simulink model "SF018A_EotProtn"  (R2013b)
settings: Solver=FixedStepDiscrete  SolverMode=SingleTasking  StartTime=0.0  StopTime=0.002  FixedStep=.002  RelTol=1e-3
undefined symbols (not defined in the file): ALLSPDDAMPG_CNT_U08, ALLSPDGAIN_CNT_U08, ARCHGLBPRM_2MILLISEC_SEC_F32, DISTLPFILFRQ_HZ_F32, EOTDAMPGLOLIM_MOTNWTMTR_F32, EOTGAINHILIM_ULS_F32, EotProtnActvRegnBypMaxThd, EotProtnDampgSlew, EotProtnDampgVehSpdTbl, EotProtnDeltaTqThd, EotProtnDftPosn, EotProtnEntrGainVehSpdTbl, EotProtnEntrGainX, EotProtnEntrStLpFilFrq, EotProtnExitDampgY, EotProtnExitStLpFilFrq, EotProtnHwAgGain, EotProtnHwAgMax, EotProtnHwAgMin, EotProtnHwDegDampgX, EotProtnMotSpdIncptSca, EotProtnMotSpdIncptX, EotProtnMotSpdIncptY, EotProtnMotVelGain, EotProtnNormDampgY, EotProtnPosnRampStep, EotProtnRackTrvlLimrAuthyThd, EotProtnRackTrvlLimrAuthyThdLimd, EotProtnRackTrvlLimrEna, EotProtnRackTrvlLimrRng, EotProtnRackTrvlLimrRngLimd, EotProtnRackTrvlLimrVehSpdThd, EotProtnRunEotVelImpctAndSoftEndStop, EotProtnSoftEndStopAuthyThd, EotProtnSoftEndStopEna, EotProtnSoftEndStopVehSpdThd, FIRSTPTDAMPG_CNT_U08, LASTPTGAIN_CNT_U08, SOFTENDSTOPSTDI_CNT_U08, SOFTENDSTOPSTENTR_CNT_U08, SOFTENDSTOPSTEXIT_CNT_U08, SOFTENDSTOPSTNORM_CNT_U08, SYSGLBPRM_MOTTQCMDHILIM_MOTNWTMTR_F32, ZEROMOTTQCMD_MOTNWTMTR_F32
libraries: NxtrAbslt x16, FloatToFixd x14, FixdToFloat x6, Fil x5, NxtrLim x5, simulink x4, NxtrMax x4, LnrIntrpnDyn x3, NxtrSign x2, BilnrIntrpnMplXDyn x2, BilnrIntrpnMplX x1, LnrIntrpn x1
(part 5 of 5)

== system SF018A_EotProtn/EotProtn/EotProtnPer1/SoftEndStop/FildEotGain/If Action Subsystem4 ==
  In1 : Inport
  Action Port : ActionPort  ActionType=default
  CopyRight2 : Subsystem  Description=|  mask(Copyright Information){none=on}
      | Copyright info block.                                               
      |                                                                     
      | Place copyright information at the top of every subsystem in design.
      mask prompts: none "No parameters"
      mask help: Place copyright information at the top of every subsystem in design.
      mask Display:
      | NxtrConf = 'Nexteer Confidential';
      | 
      | sys = bdroot; %handle for the current model ("system")
      | first = get_param(sys,'Created');
      | if(isempty(first))
      |     first = datestr(now,'yyyy');
      | else
      |     first = first(end-3:end);  %year is last four digits
      | end
      | 
      | last = get_param(sys,'LastModifiedDate');
      | if isempty(last)
      |     last = datestr(now,'yyyy');
      | else
      |     last = last(end-3:end);
      | end
      | 
      | if strcmp(first,last)
      |     fprintf('%s -- Copyright %s Nexteer',NxtrConf,first)
      | else
      |     fprintf('%s -- %s%s- %s Nexteer',NxtrConf,char(169),first,last)
      | end
  Out1 : Outport
  wires:
  In1/1 -> Out1/1

== system SF018A_EotProtn/EotProtn/EotProtnPer1/SoftEndStop/FildEotGain/If Action Subsystem5 ==
  In1 : Inport
  Action Port : ActionPort  ActionType=case
  CopyRight2 : Subsystem  Description=|  mask(Copyright Information){none=on}
      | Copyright info block.                                               
      |                                                                     
      | Place copyright information at the top of every subsystem in design.
      mask prompts: none "No parameters"
      mask help: Place copyright information at the top of every subsystem in design.
      mask Display:
      | NxtrConf = 'Nexteer Confidential';
      | 
      | sys = bdroot; %handle for the current model ("system")
      | first = get_param(sys,'Created');
      | if(isempty(first))
      |     first = datestr(now,'yyyy');
      | else
      |     first = first(end-3:end);  %year is last four digits
      | end
      | 
      | last = get_param(sys,'LastModifiedDate');
      | if isempty(last)
      |     last = datestr(now,'yyyy');
      | else
      |     last = last(end-3:end);
      | end
      | 
      | if strcmp(first,last)
      |     fprintf('%s -- Copyright %s Nexteer',NxtrConf,first)
      | else
      |     fprintf('%s -- %s%s- %s Nexteer',NxtrConf,char(169),first,last)
      | end
  Out1 : Outport
  wires:
  In1/1 -> Out1/1

== system SF018A_EotProtn/EotProtn/EotProtnPer1/SoftEndStop/If Action Subsystem2/CopyRight2 ==

== system SF018A_EotProtn/EotProtn/EotProtnPer1/SoftEndStop/If Action Subsystem4/CopyRight2 ==

== system SF018A_EotProtn/EotProtn/EotProtnPer1/SoftEndStop/LimPosnDetd/CopyRight2 ==

== system SF018A_EotProtn/EotProtn/EotProtnPer1/SoftEndStop/LimPosnDetd/If Action Subsystem ==
  In1 : Inport
  Action Port : ActionPort  ActionType=else
  CopyRight2 : Subsystem  Description=|  mask(Copyright Information){none=on}
      | Copyright info block.                                               
      |                                                                     
      | Place copyright information at the top of every subsystem in design.
      mask prompts: none "No parameters"
      mask help: Place copyright information at the top of every subsystem in design.
      mask Display:
      | NxtrConf = 'Nexteer Confidential';
      | 
      | sys = bdroot; %handle for the current model ("system")
      | first = get_param(sys,'Created');
      | if(isempty(first))
      |     first = datestr(now,'yyyy');
      | else
      |     first = first(end-3:end);  %year is last four digits
      | end
      | 
      | last = get_param(sys,'LastModifiedDate');
      | if isempty(last)
      |     last = datestr(now,'yyyy');
      | else
      |     last = last(end-3:end);
      | end
      | 
      | if strcmp(first,last)
      |     fprintf('%s -- Copyright %s Nexteer',NxtrConf,first)
      | else
      |     fprintf('%s -- %s%s- %s Nexteer',NxtrConf,char(169),first,last)
      | end
  Out1 : Outport
  wires:
  In1/1 -> Out1/1

== system SF018A_EotProtn/EotProtn/EotProtnPer1/SoftEndStop/LimPosnDetd/If Action Subsystem1 ==
  In1 : Inport
  Action Port : ActionPort  ActionType=then
  CopyRight2 : Subsystem  Description=|  mask(Copyright Information){none=on}
      | Copyright info block.                                               
      |                                                                     
      | Place copyright information at the top of every subsystem in design.
      mask prompts: none "No parameters"
      mask help: Place copyright information at the top of every subsystem in design.
      mask Display:
      | NxtrConf = 'Nexteer Confidential';
      | 
      | sys = bdroot; %handle for the current model ("system")
      | first = get_param(sys,'Created');
      | if(isempty(first))
      |     first = datestr(now,'yyyy');
      | else
      |     first = first(end-3:end);  %year is last four digits
      | end
      | 
      | last = get_param(sys,'LastModifiedDate');
      | if isempty(last)
      |     last = datestr(now,'yyyy');
      | else
      |     last = last(end-3:end);
      | end
      | 
      | if strcmp(first,last)
      |     fprintf('%s -- Copyright %s Nexteer',NxtrConf,first)
      | else
      |     fprintf('%s -- %s%s- %s Nexteer',NxtrConf,char(169),first,last)
      | end
  Out1 : Outport
  wires:
  In1/1 -> Out1/1

== system SF018A_EotProtn/EotProtn/EotProtnPer1/SoftEndStop/LimPosnDetd/If Action Subsystem2 ==
  In1 : Inport
  Action Port : ActionPort  ActionType=else
  CopyRight2 : Subsystem  Description=|  mask(Copyright Information){none=on}
      | Copyright info block.                                               
      |                                                                     
      | Place copyright information at the top of every subsystem in design.
      mask prompts: none "No parameters"
      mask help: Place copyright information at the top of every subsystem in design.
      mask Display:
      | NxtrConf = 'Nexteer Confidential';
      | 
      | sys = bdroot; %handle for the current model ("system")
      | first = get_param(sys,'Created');
      | if(isempty(first))
      |     first = datestr(now,'yyyy');
      | else
      |     first = first(end-3:end);  %year is last four digits
      | end
      | 
      | last = get_param(sys,'LastModifiedDate');
      | if isempty(last)
      |     last = datestr(now,'yyyy');
      | else
      |     last = last(end-3:end);
      | end
      | 
      | if strcmp(first,last)
      |     fprintf('%s -- Copyright %s Nexteer',NxtrConf,first)
      | else
      |     fprintf('%s -- %s%s- %s Nexteer',NxtrConf,char(169),first,last)
      | end
  Out1 : Outport
  wires:
  In1/1 -> Out1/1

== system SF018A_EotProtn/EotProtn/EotProtnPer1/SoftEndStop/LimPosnDetd/If Action Subsystem3 ==
  In1 : Inport
  Action Port : ActionPort  ActionType=then
  CopyRight2 : Subsystem  Description=|  mask(Copyright Information){none=on}
      | Copyright info block.                                               
      |                                                                     
      | Place copyright information at the top of every subsystem in design.
      mask prompts: none "No parameters"
      mask help: Place copyright information at the top of every subsystem in design.
      mask Display:
      | NxtrConf = 'Nexteer Confidential';
      | 
      | sys = bdroot; %handle for the current model ("system")
      | first = get_param(sys,'Created');
      | if(isempty(first))
      |     first = datestr(now,'yyyy');
      | else
      |     first = first(end-3:end);  %year is last four digits
      | end
      | 
      | last = get_param(sys,'LastModifiedDate');
      | if isempty(last)
      |     last = datestr(now,'yyyy');
      | else
      |     last = last(end-3:end);
      | end
      | 
      | if strcmp(first,last)
      |     fprintf('%s -- Copyright %s Nexteer',NxtrConf,first)
      | else
      |     fprintf('%s -- %s%s- %s Nexteer',NxtrConf,char(169),first,last)
      | end
  Out1 : Outport
  wires:
  In1/1 -> Out1/1

== system SF018A_EotProtn/EotProtn/EotProtnPer1/SoftEndStop/LimPosnDetd/If Action Subsystem4 ==
  In1 : Inport
  Action Port : ActionPort  ActionType=else
  CopyRight2 : Subsystem  Description=|  mask(Copyright Information){none=on}
      | Copyright info block.                                               
      |                                                                     
      | Place copyright information at the top of every subsystem in design.
      mask prompts: none "No parameters"
      mask help: Place copyright information at the top of every subsystem in design.
      mask Display:
      | NxtrConf = 'Nexteer Confidential';
      | 
      | sys = bdroot; %handle for the current model ("system")
      | first = get_param(sys,'Created');
      | if(isempty(first))
      |     first = datestr(now,'yyyy');
      | else
      |     first = first(end-3:end);  %year is last four digits
      | end
      | 
      | last = get_param(sys,'LastModifiedDate');
      | if isempty(last)
      |     last = datestr(now,'yyyy');
      | else
      |     last = last(end-3:end);
      | end
      | 
      | if strcmp(first,last)
      |     fprintf('%s -- Copyright %s Nexteer',NxtrConf,first)
      | else
      |     fprintf('%s -- %s%s- %s Nexteer',NxtrConf,char(169),first,last)
      | end
  Out1 : Outport
  wires:
  In1/1 -> Out1/1

== system SF018A_EotProtn/EotProtn/EotProtnPer1/SoftEndStop/LimPosnDetd/If Action Subsystem5 ==
  In1 : Inport
  Action Port : ActionPort  ActionType=then
  CopyRight2 : Subsystem  Description=|  mask(Copyright Information){none=on}
      | Copyright info block.                                               
      |                                                                     
      | Place copyright information at the top of every subsystem in design.
      mask prompts: none "No parameters"
      mask help: Place copyright information at the top of every subsystem in design.
      mask Display:
      | NxtrConf = 'Nexteer Confidential';
      | 
      | sys = bdroot; %handle for the current model ("system")
      | first = get_param(sys,'Created');
      | if(isempty(first))
      |     first = datestr(now,'yyyy');
      | else
      |     first = first(end-3:end);  %year is last four digits
      | end
      | 
      | last = get_param(sys,'LastModifiedDate');
      | if isempty(last)
      |     last = datestr(now,'yyyy');
      | else
      |     last = last(end-3:end);
      | end
      | 
      | if strcmp(first,last)
      |     fprintf('%s -- Copyright %s Nexteer',NxtrConf,first)
      | else
      |     fprintf('%s -- %s%s- %s Nexteer',NxtrConf,char(169),first,last)
      | end
  Out1 : Outport
  wires:
  In1/1 -> Out1/1

== system SF018A_EotProtn/EotProtn/EotProtnPer1/SoftEndStop/LimPosnDetd/If Action Subsystem6 ==
  In1 : Inport
  Action Port : ActionPort  ActionType=then
  CopyRight2 : Subsystem  Description=|  mask(Copyright Information){none=on}
      | Copyright info block.                                               
      |                                                                     
      | Place copyright information at the top of every subsystem in design.
      mask prompts: none "No parameters"
      mask help: Place copyright information at the top of every subsystem in design.
      mask Display:
      | NxtrConf = 'Nexteer Confidential';
      | 
      | sys = bdroot; %handle for the current model ("system")
      | first = get_param(sys,'Created');
      | if(isempty(first))
      |     first = datestr(now,'yyyy');
      | else
      |     first = first(end-3:end);  %year is last four digits
      | end
      | 
      | last = get_param(sys,'LastModifiedDate');
      | if isempty(last)
      |     last = datestr(now,'yyyy');
      | else
      |     last = last(end-3:end);
      | end
      | 
      | if strcmp(first,last)
      |     fprintf('%s -- Copyright %s Nexteer',NxtrConf,first)
      | else
      |     fprintf('%s -- %s%s- %s Nexteer',NxtrConf,char(169),first,last)
      | end
  Out1 : Outport
  wires:
  In1/1 -> Out1/1

== system SF018A_EotProtn/EotProtn/EotProtnPer1/SoftEndStop/LimPosnDetd/If Action Subsystem7 ==
  In1 : Inport
  Action Port : ActionPort  ActionType=else
  CopyRight2 : Subsystem  Description=|  mask(Copyright Information){none=on}
      | Copyright info block.                                               
      |                                                                     
      | Place copyright information at the top of every subsystem in design.
      mask prompts: none "No parameters"
      mask help: Place copyright information at the top of every subsystem in design.
      mask Display:
      | NxtrConf = 'Nexteer Confidential';
      | 
      | sys = bdroot; %handle for the current model ("system")
      | first = get_param(sys,'Created');
      | if(isempty(first))
      |     first = datestr(now,'yyyy');
      | else
      |     first = first(end-3:end);  %year is last four digits
      | end
      | 
      | last = get_param(sys,'LastModifiedDate');
      | if isempty(last)
      |     last = datestr(now,'yyyy');
      | else
      |     last = last(end-3:end);
      | end
      | 
      | if strcmp(first,last)
      |     fprintf('%s -- Copyright %s Nexteer',NxtrConf,first)
      | else
      |     fprintf('%s -- %s%s- %s Nexteer',NxtrConf,char(169),first,last)
      | end
  Out1 : Outport
  wires:
  In1/1 -> Out1/1

== system SF018A_EotProtn/EotProtn/EotProtnPer1/SoftEndStop/PosnCtrl/CopyRight2 ==

== system SF018A_EotProtn/EotProtn/EotProtnPer1/SoftEndStop/PosnCtrl/If Action Subsystem ==
  In1 : Inport
  Action Port : ActionPort  ActionType=else
  CopyRight2 : Subsystem  Description=|  mask(Copyright Information){none=on}
      | Copyright info block.                                               
      |                                                                     
      | Place copyright information at the top of every subsystem in design.
      mask prompts: none "No parameters"
      mask help: Place copyright information at the top of every subsystem in design.
      mask Display:
      | NxtrConf = 'Nexteer Confidential';
      | 
      | sys = bdroot; %handle for the current model ("system")
      | first = get_param(sys,'Created');
      | if(isempty(first))
      |     first = datestr(now,'yyyy');
      | else
      |     first = first(end-3:end);  %year is last four digits
      | end
      | 
      | last = get_param(sys,'LastModifiedDate');
      | if isempty(last)
      |     last = datestr(now,'yyyy');
      | else
      |     last = last(end-3:end);
      | end
      | 
      | if strcmp(first,last)
      |     fprintf('%s -- Copyright %s Nexteer',NxtrConf,first)
      | else
      |     fprintf('%s -- %s%s- %s Nexteer',NxtrConf,char(169),first,last)
      | end
  Out1 : Outport
  wires:
  In1/1 -> Out1/1

== system SF018A_EotProtn/EotProtn/EotProtnPer1/SoftEndStop/PosnCtrl/If Action Subsystem1 ==
  In1 : Inport
  Action Port : ActionPort  ActionType=then
  CopyRight2 : Subsystem  Description=|  mask(Copyright Information){none=on}
      | Copyright info block.                                               
      |                                                                     
      | Place copyright information at the top of every subsystem in design.
      mask prompts: none "No parameters"
      mask help: Place copyright information at the top of every subsystem in design.
      mask Display:
      | NxtrConf = 'Nexteer Confidential';
      | 
      | sys = bdroot; %handle for the current model ("system")
      | first = get_param(sys,'Created');
      | if(isempty(first))
      |     first = datestr(now,'yyyy');
      | else
      |     first = first(end-3:end);  %year is last four digits
      | end
      | 
      | last = get_param(sys,'LastModifiedDate');
      | if isempty(last)
      |     last = datestr(now,'yyyy');
      | else
      |     last = last(end-3:end);
      | end
      | 
      | if strcmp(first,last)
      |     fprintf('%s -- Copyright %s Nexteer',NxtrConf,first)
      | else
      |     fprintf('%s -- %s%s- %s Nexteer',NxtrConf,char(169),first,last)
      | end
  Out1 : Outport
  wires:
  In1/1 -> Out1/1

== system SF018A_EotProtn/EotProtn/EotProtnPer1/SoftEndStop/RackTrvlLimrDi/CopyRight2 ==

== system SF018A_EotProtn/EotProtn/EotProtnPer1/SoftEndStop/RackTrvlLimrInin/CopyRight2 ==

== system SF018A_EotProtn/EotProtn/EotProtnPer1/SoftEndStop/RackTrvlLimrInin/If Action Subsystem ==
  Action Port : ActionPort  ActionType=then
  Constant : Constant  RequirementInfo={'linktype_rmi_doors' '0000ba56 (/E-STEER Core/SubSystem Specifications/Application Functions/SF018A End-of-Travel Actuator Management- EOT Impact and Soft Stops)' '#SF018A_129' 'true' 'REQ: SF018A_129' '' } %GIDa_6618d1ea_ce4f_4376_9ab5_a20895642902  Value=true
  CopyRight2 : Subsystem  Description=|  mask(Copyright Information){none=on}
      | Copyright info block.                                               
      |                                                                     
      | Place copyright information at the top of every subsystem in design.
      mask prompts: none "No parameters"
      mask help: Place copyright information at the top of every subsystem in design.
      mask Display:
      | NxtrConf = 'Nexteer Confidential';
      | 
      | sys = bdroot; %handle for the current model ("system")
      | first = get_param(sys,'Created');
      | if(isempty(first))
      |     first = datestr(now,'yyyy');
      | else
      |     first = first(end-3:end);  %year is last four digits
      | end
      | 
      | last = get_param(sys,'LastModifiedDate');
      | if isempty(last)
      |     last = datestr(now,'yyyy');
      | else
      |     last = last(end-3:end);
      | end
      | 
      | if strcmp(first,last)
      |     fprintf('%s -- Copyright %s Nexteer',NxtrConf,first)
      | else
      |     fprintf('%s -- %s%s- %s Nexteer',NxtrConf,char(169),first,last)
      | end
  true : Outport
  wires:
  Constant/1 -> true/1

== system SF018A_EotProtn/EotProtn/EotProtnPer1/SoftEndStop/RackTrvlLimrInin/If Action Subsystem1 ==
  Action Port : ActionPort  ActionType=elseif
  Constant : Constant  RequirementInfo={'linktype_rmi_doors' '0000ba56 (/E-STEER Core/SubSystem Specifications/Application Functions/SF018A End-of-Travel Actuator Management- EOT Impact and Soft Stops)' '#SF018A_124' 'true' 'REQ: SF018A_124' '' } %GIDa_694fcd67_0597_4d08_9ac1_2ea4c0af129e  Value=false
  CopyRight2 : Subsystem  Description=|  mask(Copyright Information){none=on}
      | Copyright info block.                                               
      |                                                                     
      | Place copyright information at the top of every subsystem in design.
      mask prompts: none "No parameters"
      mask help: Place copyright information at the top of every subsystem in design.
      mask Display:
      | NxtrConf = 'Nexteer Confidential';
      | 
      | sys = bdroot; %handle for the current model ("system")
      | first = get_param(sys,'Created');
      | if(isempty(first))
      |     first = datestr(now,'yyyy');
      | else
      |     first = first(end-3:end);  %year is last four digits
      | end
      | 
      | last = get_param(sys,'LastModifiedDate');
      | if isempty(last)
      |     last = datestr(now,'yyyy');
      | else
      |     last = last(end-3:end);
      | end
      | 
      | if strcmp(first,last)
      |     fprintf('%s -- Copyright %s Nexteer',NxtrConf,first)
      | else
      |     fprintf('%s -- %s%s- %s Nexteer',NxtrConf,char(169),first,last)
      | end
  false : Outport
  wires:
  Constant/1 -> false/1

== system SF018A_EotProtn/EotProtn/EotProtnPer1/SoftEndStop/RackTrvlLimrInin/If Action Subsystem2 ==
  In1 : Inport
  Action Port : ActionPort  ActionType=else
  CopyRight2 : Subsystem  Description=|  mask(Copyright Information){none=on}
      | Copyright info block.                                               
      |                                                                     
      | Place copyright information at the top of every subsystem in design.
      mask prompts: none "No parameters"
      mask help: Place copyright information at the top of every subsystem in design.
      mask Display:
      | NxtrConf = 'Nexteer Confidential';
      | 
      | sys = bdroot; %handle for the current model ("system")
      | first = get_param(sys,'Created');
      | if(isempty(first))
      |     first = datestr(now,'yyyy');
      | else
      |     first = first(end-3:end);  %year is last four digits
      | end
      | 
      | last = get_param(sys,'LastModifiedDate');
      | if isempty(last)
      |     last = datestr(now,'yyyy');
      | else
      |     last = last(end-3:end);
      | end
      | 
      | if strcmp(first,last)
      |     fprintf('%s -- Copyright %s Nexteer',NxtrConf,first)
      | else
      |     fprintf('%s -- %s%s- %s Nexteer',NxtrConf,char(169),first,last)
      | end
  Out1 : Outport
  wires:
  In1/1 -> Out1/1

== system SF018A_EotProtn/EotProtn/EotProtnPer1/SoftEndStopStCtrl/Keep State/CopyRight2 ==

== system SF018A_EotProtn/EotProtn/EotProtnPer1/SoftEndStopStCtrl/PriorityVec1/CopyRight2 ==

== system SF018A_EotProtn/EotProtn/EotProtnPer1/SoftEndStopStCtrl/PriorityVec2/CopyRight2 ==

== system SF018A_EotProtn/EotProtn/EotProtnPer1/SoftEndStopStCtrl/PriorityVec3/CopyRight2 ==

== system SF018A_EotProtn/EotProtn/EotProtnPer1/SoftEndStopStCtrl/PriorityVec4/CopyRight2 ==

== system SF018A_EotProtn/EotProtn/EotProtnPer1/EotVelImpct/Ramp/If Action Subsystem/CopyRight2 ==

== system SF018A_EotProtn/EotProtn/EotProtnPer1/EotVelImpct/Ramp/If Action Subsystem1/CopyRight2 ==

== system SF018A_EotProtn/EotProtn/EotProtnPer1/SoftEndStop/CalcEntrGain/If Action Subsystem/CopyRight2 ==

== system SF018A_EotProtn/EotProtn/EotProtnPer1/SoftEndStop/CalcEntrGain/If Action Subsystem1/CopyRight2 ==

== system SF018A_EotProtn/EotProtn/EotProtnPer1/SoftEndStop/CalcEotDampg/ Disabled/CopyRight2 ==

== system SF018A_EotProtn/EotProtn/EotProtnPer1/SoftEndStop/CalcEotDampg/ Exiting/CopyRight2 ==

== system SF018A_EotProtn/EotProtn/EotProtnPer1/SoftEndStop/CalcEotDampg/ Normal OR Entering/CopyRight2 ==

== system SF018A_EotProtn/EotProtn/EotProtnPer1/SoftEndStop/CalcEotDampg/If Action Subsystem/CopyRight2 ==

== system SF018A_EotProtn/EotProtn/EotProtnPer1/SoftEndStop/CalcEotDampg/If Action Subsystem1/CopyRight2 ==

== system SF018A_EotProtn/EotProtn/EotProtnPer1/SoftEndStop/CalcEotGain/ Disabled/CopyRight2 ==

== system SF018A_EotProtn/EotProtn/EotProtnPer1/SoftEndStop/CalcEotGain/ Exiting/CopyRight2 ==

== system SF018A_EotProtn/EotProtn/EotProtnPer1/SoftEndStop/CalcEotGain/Entering or Normal/CopyRight2 ==

== system SF018A_EotProtn/EotProtn/EotProtnPer1/SoftEndStop/FildEotGain/If Action Subsystem3/CopyRight2 ==

== system SF018A_EotProtn/EotProtn/EotProtnPer1/SoftEndStop/FildEotGain/If Action Subsystem4/CopyRight2 ==

== system SF018A_EotProtn/EotProtn/EotProtnPer1/SoftEndStop/FildEotGain/If Action Subsystem5/CopyRight2 ==

== system SF018A_EotProtn/EotProtn/EotProtnPer1/SoftEndStop/LimPosnDetd/If Action Subsystem/CopyRight2 ==

== system SF018A_EotProtn/EotProtn/EotProtnPer1/SoftEndStop/LimPosnDetd/If Action Subsystem1/CopyRight2 ==

== system SF018A_EotProtn/EotProtn/EotProtnPer1/SoftEndStop/LimPosnDetd/If Action Subsystem2/CopyRight2 ==

== system SF018A_EotProtn/EotProtn/EotProtnPer1/SoftEndStop/LimPosnDetd/If Action Subsystem3/CopyRight2 ==

== system SF018A_EotProtn/EotProtn/EotProtnPer1/SoftEndStop/LimPosnDetd/If Action Subsystem4/CopyRight2 ==

== system SF018A_EotProtn/EotProtn/EotProtnPer1/SoftEndStop/LimPosnDetd/If Action Subsystem5/CopyRight2 ==

== system SF018A_EotProtn/EotProtn/EotProtnPer1/SoftEndStop/LimPosnDetd/If Action Subsystem6/CopyRight2 ==

== system SF018A_EotProtn/EotProtn/EotProtnPer1/SoftEndStop/LimPosnDetd/If Action Subsystem7/CopyRight2 ==

== system SF018A_EotProtn/EotProtn/EotProtnPer1/SoftEndStop/PosnCtrl/If Action Subsystem/CopyRight2 ==

== system SF018A_EotProtn/EotProtn/EotProtnPer1/SoftEndStop/PosnCtrl/If Action Subsystem1/CopyRight2 ==

== system SF018A_EotProtn/EotProtn/EotProtnPer1/SoftEndStop/RackTrvlLimrInin/If Action Subsystem/CopyRight2 ==

== system SF018A_EotProtn/EotProtn/EotProtnPer1/SoftEndStop/RackTrvlLimrInin/If Action Subsystem1/CopyRight2 ==

== system SF018A_EotProtn/EotProtn/EotProtnPer1/SoftEndStop/RackTrvlLimrInin/If Action Subsystem2/CopyRight2 ==
